simulink model "GUI_V4"  (Simulink 7.7)
settings: Solver=FixedStepDiscrete  SolverMode=SingleTasking  StartTime=0.0  StopTime=60*60*24*365  FixedStep=0.001  RelTol=1e-3
libraries: Diamond16AT_UNAL x2, simulink x1
settings Model: Creator=crist  LastModifiedBy=crist  SimulationMode=external  BufferReuse=off
settings OptimizationCC: BlockReduction=off  OptimizeBlockIOStorage=off  BufferReuse=off  ExpressionFolding=off  LocalBlockOutputs=off
settings HardwareCC: ProdIntDivRoundTo=Zero  ProdEndianess=LittleEndian  ProdHWDeviceType=Generic->32-bit x86 compatible
settings RTWCC: SystemTargetFile=xpctarget.tlc  TemplateMakefile=xpc_default_tmf  Description=xPC Target  ProcessScript=xpctarget_make_rtw_hook  RTWCompilerOptimization=On
settings xpcTargetCC: TargetFcnLib=ansi_tfl_table_tmw.mat  TargetFunctionLibrary=XPC_BLAS  FunctionExecutionProfile=off  CodeExecutionProfiling=off  ERTCodeCoverageTool=None  ParMdlRefBuildCompliant=on  CombineSignalStateStructs=off  PortableWordSizes=off  xPCTaskExecutionProfile=off  xPCRL32EventNumber=5000  xPCLoadParamSetFile=off  xPCConcurrentTasks=off  xPCEnableSFAnimation=off

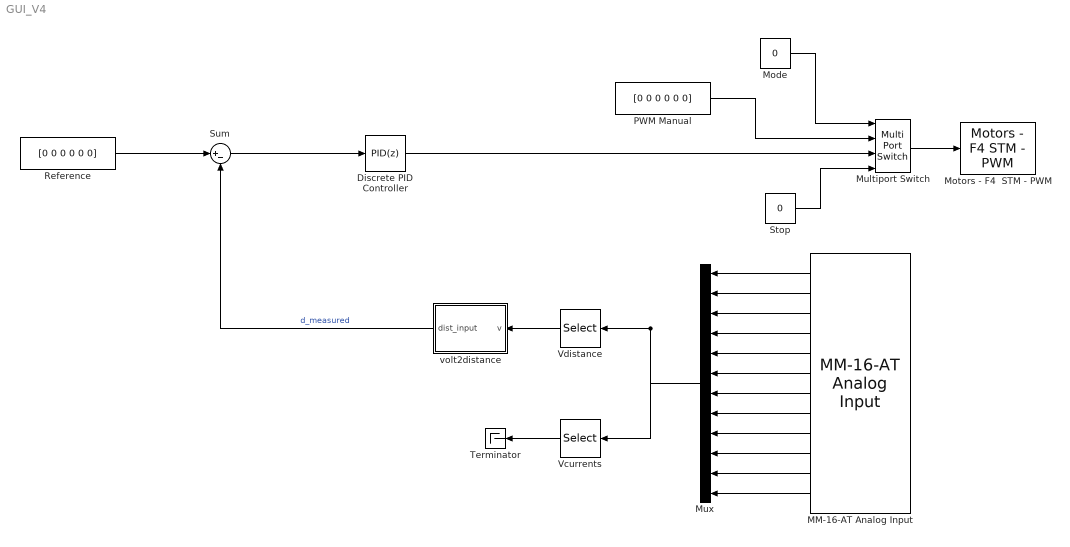
== system GUI_V4 ==
  Discrete PID Controller : simulink/Continuous/PID Controller  SystemSampleTime=-1  Controller=PID  TimeDomain=Discrete-time  SampleTime=-1  IntegratorMethod=Forward Euler  FilterMethod=Forward Euler  Form=Parallel  P=100  I=25  D=0  N=100  InitialConditionSource=internal  InitialConditionForIntegrator=0  InitialConditionForFilter=0  ExternalReset=none  LimitOutput=off  UpperSaturationLimit=inf  LowerSaturationLimit=-inf  LinearizeAsGain=off  AntiWindupMode=none  Kb=1  TrackingMode=off  Kt=1  PParamMin=[]  PParamMax=[]  IParamMin=[]  IParamMax=[]  DParamMin=[]  DParamMax=[]  NParamMin=[]  NParamMax=[]  KbParamMin=[]  KbParamMax=[]  KtParamMin=[]  KtParamMax=[]  POutMin=[]  POutMax=[]  IOutMin=[]  IOutMax=[]  DOutMin=[]  DOutMax=[]  NOutMin=[]  NOutMax=[]  KbOutMin=[]  KbOutMax=[]  KtOutMin=[]  KtOutMax=[]  IntegratorOutMin=[]  IntegratorOutMax=[]  FilterOutMin=[]  FilterOutMax=[]  SumOutMin=[]  SumOutMax=[]  SumI1OutMin=[]  SumI1OutMax=[]  SumI2OutMin=[]  SumI2OutMax=[]  SumI3OutMin=[]  SumI3OutMax=[]  SumDOutMin=[]  SumDOutMax=[]  SaturationOutMin=[]  SaturationOutMax=[]  IntegratorContinuousStateAttributes=''  IntegratorStateMustResolveToSignalObject=off  IntegratorRTWStateStorageClass=Auto  FilterContinuousStateAttributes=''  FilterStateMustResolveToSignalObject=off  FilterRTWStateStorageClass=Auto
  MM-16-AT Analog Input : Diamond16AT_UNAL/Diamond MM-16-AT/MM-16-AT Analog Input  configuration=16 Single-ended  firstChan=1  numChans=12  range=0 to 10V  sampleTime=0.001  base=300
  Mode : Constant  Value=0
  Motors - F4  STM - PWM : Diamond16AT_UNAL/PWM Generation/Motors - F4  STM - PWM  SystemSampleTime=-1  Satura=80  SamTime=0.001
  Multiport Switch : MultiPortSwitch  DataPortOrder=Specify indices  DataPortIndices={2,1,0}  DiagnosticForDefault=Warning  zeroidx=off
  Mux : Mux  Inputs=12
  PWM Manual : Constant  Value=[0 0 0 0 0 0]
  Reference : Constant  Value=[0 0 0 0 0 0]
  Stop : Constant  Value=0
  Sum : Sum  Inputs=|+-
  Terminator : Terminator
  Vcurrents : Selector  InputPortWidth=12  IndexOptions=Index vector (dialog)  Indices=[2 4 6 8 10 12]  OutputSizes=1
  Vdistance : Selector  NumberOfDimensions=2  InputPortWidth=12  IndexOptions=Index vector (dialog),Index vector (dialog)  Indices=[1 3 5 7 9 11],1  OutputSizes=1,1
  volt2distance : Stateflow chart  TreatAsAtomicUnit=on
  wires:
  Multiport Switch/1 -> Motors - F4  STM - PWM/1
  Mode/1 -> Multiport Switch/1
  Vcurrents/1 -> Terminator/1
  Vdistance/1 -> volt2distance/1(v)
  Mux/1 -> Vcurrents/1, Vdistance/1
  MM-16-AT Analog Input/12 -> Mux/12
  MM-16-AT Analog Input/11 -> Mux/11
  MM-16-AT Analog Input/10 -> Mux/10
  MM-16-AT Analog Input/9 -> Mux/9
  MM-16-AT Analog Input/8 -> Mux/8
  MM-16-AT Analog Input/7 -> Mux/7
  MM-16-AT Analog Input/6 -> Mux/6
  MM-16-AT Analog Input/5 -> Mux/5
  MM-16-AT Analog Input/4 -> Mux/4
  MM-16-AT Analog Input/3 -> Mux/3
  MM-16-AT Analog Input/2 -> Mux/2
  MM-16-AT Analog Input/1 -> Mux/1
  Discrete PID Controller/1 -> Multiport Switch/3
  Sum/1 -> Discrete PID Controller/1
  volt2distance/1(dist_input) -> Sum/2  "d_measured"
  Reference/1 -> Sum/1
  PWM Manual/1 -> Multiport Switch/2
  Stop/1 -> Multiport Switch/4

== matlab function volt2distance ==
  data: v input double; dist_input output double
function dist_input = volt2distance(v)

m=[-0.068432671	-0.06935123	-0.06993007	-0.068736142	-0.068432671	-0.068888889]';
b=[0.897373068	0.900514541	0.876083916	0.900243902	0.898741722	0.901]';

dist_input = m.*v + b;
